simulink model "que3"  (R2020b)
settings: Solver=VariableStepAuto  StartTime=0.0  StopTime=0.10  RelTol=1e-3
settings Model: Creator=ANUJA  LastModifiedBy=ANUJA

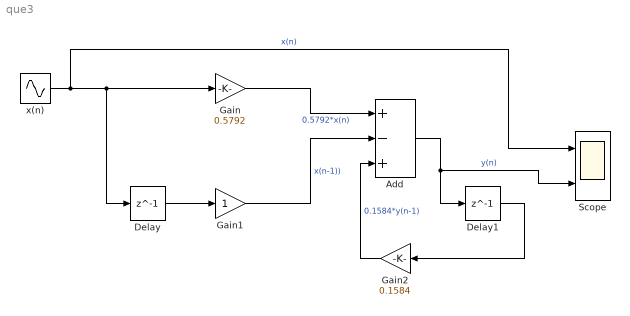
== system que3 ==
  Add : Sum  Inputs=+-+
  Delay : Delay  DelayLength=1  InitialCondition=0
  Delay1 : Delay  DelayLength=1  InitialCondition=0
  Gain : Gain  Gain=0.5792
  Gain1 : Gain
  Gain2 : Gain  Gain=0.1584
  Scope : Scope  NumInputPorts=2
  x(n) : Sin  Frequency=2*3.14*950  SampleTime=0
  wires:
  x(n)/1 -> Scope/1, Gain/1, Delay/1  "x(n)"
  Delay/1 -> Gain1/1
  Gain/1 -> Add/1  "0.5792*x(n)"
  Gain1/1 -> Add/2  "x(n-1))"
  Gain2/1 -> Add/3  "0.1584*y(n-1)"
  Delay1/1 -> Gain2/1
  Add/1 -> Scope/2, Delay1/1  "y(n)"
